simulink model "TIM_5_1_2"  (R2022b)
settings: Solver=VariableStepAuto  StartTime=0.0  StopTime=2  RelTol=1e-3
(part 4 of 4)

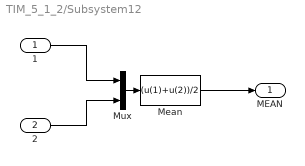
== system TIM_5_1_2/Subsystem12 ==
  1 : Inport
  2 : Inport  Port=2
  Mean : Fcn  Expr=(u(1)+u(2))/2
  Mux : Mux  Inputs=2
  MEAN : Outport  VectorParamsAs1DForOutWhenUnconnected=off
  wires:
  1/1 -> Mux/1
  Mux/1 -> Mean/1
  2/1 -> Mux/2
  Mean/1 -> MEAN/1

== matlab function TIM_5_1_2/media ==
  data: u input; y output
function y = media(u)

y = mean(u);

== matlab function TIM_5_1_2/media2 ==
  data: u input; y output
function y = media(u)

y = mean(u);

== matlab function TIM_5_1_2/media3 ==
  data: u input; y output
function y = media(u)

y = mean(u);

== matlab function TIM_5_1_2/media4 ==
  data: u input; y output
function y = media(u)

y = mean(u);

== matlab function TIM_5_1_2/media5 ==
  data: u input; y output
function y = media(u)

y = mean(u);

== matlab function TIM_5_1_2/media6 ==
  data: u input; y output
function y = media(u)

y = mean(u);

== matlab function TIM_5_1_2/media7 ==
  data: u input; y output
function y = media(u)

y = mean(u);

== matlab function TIM_5_1_2/media8 ==
  data: u input; y output
function y = media(u)

y = mean(u);

== matlab function TIM_5_1_2/media1 ==
  data: u input; y output
function y = media(u)

y = mean(u);

== matlab function TIM_5_1_2/media9 ==
  data: u input; y output
function y = media(u)

y = mean(u);

== matlab function TIM_5_1_2/media10 ==
  data: u input; y output
function y = media(u)

y = mean(u);

== matlab function TIM_5_1_2/media11 ==
  data: u input; y output
function y = media(u)

y = mean(u);

== matlab function TIM_5_1_2/media12 ==
  data: u input; y output
function y = media(u)

y = mean(u);

== matlab function TIM_5_1_2/media13 ==
  data: u input; y output
function y = media(u)

y = mean(u);
